simulink model "FIR_Filter"  (R2020b)
settings: Solver=VariableStepAuto  StartTime=0.0  StopTime=10.0  RelTol=1e-3
values from neighbouring files (symbols this model uses):
  a = 2    [data.mat]
  b = 3    [data.mat]
  c = 4    [data.mat]
  d = 5    [data.mat]
settings Model: Creator=vijay jagtap  LastModifiedBy=vijay jagtap

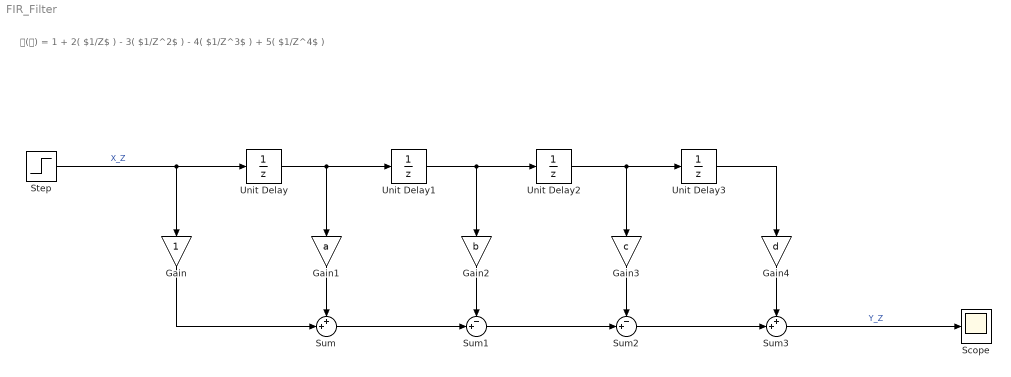
== system FIR_Filter ==
  note: 𝐇(𝐳) = 1 + 2( $1/Z$ ) - 3( $1/Z^2$ ) - 4( $1/Z^3$ ) + 5( $1/Z^4$ )
  Gain : Gain
  Gain1 : Gain  Gain=a
  Gain2 : Gain  Gain=b
  Gain3 : Gain  Gain=c
  Gain4 : Gain  Gain=d
  Scope : Scope
  Step : Step  After=5  SampleTime=0
  Sum : Sum  Inputs=++|
  Sum1 : Sum  Inputs=-+|
  Sum2 : Sum  Inputs=-+|
  Sum3 : Sum  Inputs=++|
  Unit Delay{,1..3} (4 alike) : UnitDelay  SampleTime=-1  HasFrameUpgradeWarning=on
  wires:
  Step/1 -> Unit Delay/1, Gain/1  "X_Z"
  Unit Delay/1 -> Gain1/1, Unit Delay1/1
  Unit Delay1/1 -> Unit Delay2/1, Gain2/1
  Unit Delay2/1 -> Unit Delay3/1, Gain3/1
  Unit Delay3/1 -> Gain4/1
  Gain1/1 -> Sum/1
  Gain/1 -> Sum/2
  Sum2/1 -> Sum3/2
  Gain4/1 -> Sum3/1
  Gain3/1 -> Sum2/1
  Sum1/1 -> Sum2/2
  Gain2/1 -> Sum1/1
  Sum/1 -> Sum1/2
  Sum3/1 -> Scope/1  "Y_Z"
